simulink model "Two_Zone_MVDC_12pulse_ACDC_degradation"  (R2020b)
settings: Solver=FixedStepAuto  StartTime=0.0  StopTime=40  FixedStep=TsELEC  MaxStep=1  RelTol=1e-3  EnableMultiTasking=on
InitFcn:
  | TsELEC = 1e-4;
  | Ts = 1e-4;
undefined symbols (not defined in the file): DiscIntNeverNeededParam, droop1, droop2, GABDA, GABDB, GBBDA, GBBDB, GPMMA, GPPMB, GPPMC, SADA, SADB, SADC, SADD, SBDA, SBDB, SBDC, SCDA, SCDB, SCDC, SCDD, SDDA, SDDB, SDDC, SDDD, SDDE
libraries: fl_lib x92, nesl_utility x49, ee_lib x36, powerlib x1, simulink x1
(part 3 of 3)

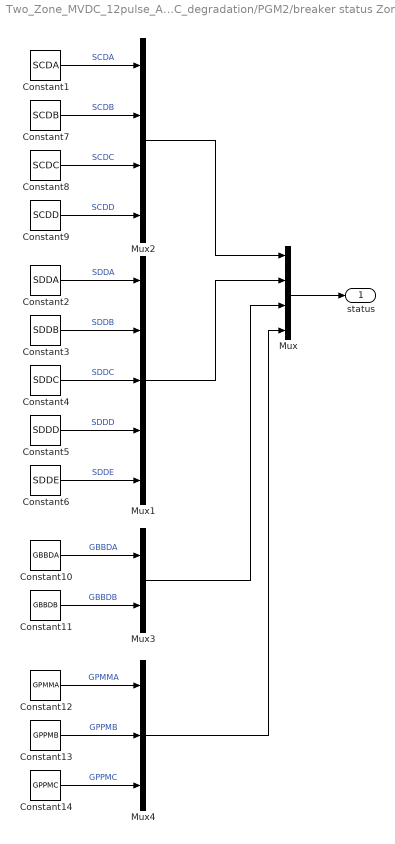
== system Two_Zone_MVDC_12pulse_ACDC_degradation/PGM2/breaker status Zone 2 ==
  Constant1 : Constant  Value=SCDA  SampleTime=Ts
  Constant10 : Constant  Value=GBBDA  SampleTime=Ts
  Constant11 : Constant  Value=GBBDB  SampleTime=Ts
  Constant12 : Constant  Value=GPMMA  SampleTime=Ts
  Constant13 : Constant  Value=GPPMB  SampleTime=Ts
  Constant14 : Constant  Value=GPPMC  SampleTime=Ts
  Constant2 : Constant  Value=SDDA  SampleTime=Ts
  Constant3 : Constant  Value=SDDB  SampleTime=Ts
  Constant4 : Constant  Value=SDDC  VectorParams1D=off  SampleTime=Ts
  Constant5 : Constant  Value=SDDD  SampleTime=Ts
  Constant6 : Constant  Value=SDDE  SampleTime=Ts
  Constant7 : Constant  Value=SCDB  SampleTime=Ts
  Constant8 : Constant  Value=SCDC  SampleTime=Ts
  Constant9 : Constant  Value=SCDD  SampleTime=Ts
  Mux : Mux  Inputs=[4 5 2 3]
  Mux1 : Mux  Inputs=5
  Mux2 : Mux
  Mux3 : Mux  Inputs=2
  Mux4 : Mux  Inputs=3
  status : Outport  VectorParamsAs1DForOutWhenUnconnected=off
  wires:
  Mux/1 -> status/1
  Constant9/1 -> Mux2/4  "SCDD"
  Constant8/1 -> Mux2/3  "SCDC"
  Constant7/1 -> Mux2/2  "SCDB"
  Constant1/1 -> Mux2/1  "SCDA"
  Constant6/1 -> Mux1/5  "SDDE"
  Constant4/1 -> Mux1/3  "SDDC"
  Constant3/1 -> Mux1/2  "SDDB"
  Constant2/1 -> Mux1/1  "SDDA"
  Constant5/1 -> Mux1/4  "SDDD"
  Constant10/1 -> Mux3/1  "GBBDA"
  Constant11/1 -> Mux3/2  "GBBDB"
  Constant12/1 -> Mux4/1  "GPMMA"
  Constant13/1 -> Mux4/2  "GPPMB"
  Constant14/1 -> Mux4/3  "GPPMC"
  Mux2/1 -> Mux/1
  Mux1/1 -> Mux/2
  Mux3/1 -> Mux/3
  Mux4/1 -> Mux/4

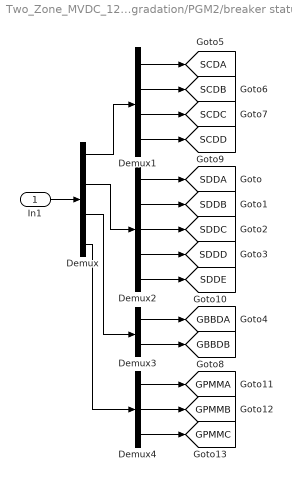
== system Two_Zone_MVDC_12pulse_ACDC_degradation/PGM2/breaker status1 ==
  In1 : Inport
  Demux : Demux  Outputs=[4 5 2 3]
  Demux1 : Demux
  Demux2 : Demux  Outputs=5
  Demux3 : Demux  Outputs=2
  Demux4 : Demux  Outputs=3
  tag scope: GBBDA=global, GBBDB=global, GPMMA=global, GPMMB=global, GPMMC=global, SCDA=global, SCDB=global, SCDC=global, SCDD=global, SDDA=global, SDDB=global, SDDC=global, SDDD=global, SDDE=global
  wires:
  Demux/4 -> Demux4/1
  Demux4/3 -> [GPMMC]
  Demux4/2 -> [GPMMB]
  Demux4/1 -> [GPMMA]
  Demux/3 -> Demux3/1
  Demux3/2 -> [GBBDB]
  Demux3/1 -> [GBBDA]
  Demux/2 -> Demux2/1
  Demux/1 -> Demux1/1
  Demux2/5 -> [SDDE]
  Demux1/4 -> [SCDD]
  Demux1/3 -> [SCDC]
  Demux1/2 -> [SCDB]
  Demux1/1 -> [SCDA]
  In1/1 -> Demux/1
  Demux2/4 -> [SDDD]
  Demux2/3 -> [SDDC]
  Demux2/1 -> [SDDA]
  Demux2/2 -> [SDDB]

== system Two_Zone_MVDC_12pulse_ACDC_degradation/PGM2/voltage droop ==
  droop : Inport
  voltage : Inport  Port=2
  Discrete-Time Integrator : DiscreteIntegrator  gainval=10  InitialCondition=0.9  SampleTime=-1  ICPrevOutput=DiscIntNeverNeededParam  ICPrevScaledInput=DiscIntNeverNeededParam
  Simulink-PS Converter : nesl_utility/Simulink-PS Converter  PhysicalDomain=network_engine_domain  SubClassName=ps_input  LeftPortType=input  RightPortType=output  PseudoPeriodic=off  Frequencies=[]  NoiseDistribution=none  NoiseParameters=[]  Unit=1  AffineConversion=off  FilteringAndDerivatives=provide  SimscapeFilterOrder=1  InputFilterTimeConstant=0.001  UdotUserProvided=0
  Sum : Sum  Inputs=|+-
  Sum1 : Sum  Inputs=|+-
  Vref : Constant
  output : PMIOPort  Side=Right
  wires:
  voltage/1 -> Sum1/2
  Sum1/1 -> Discrete-Time Integrator/1
  Vref/1 -> Sum/1
  droop/1 -> Sum/2
  Sum/1 -> Sum1/1
  Discrete-Time Integrator/1 -> Simulink-PS Converter/1
  connections:
  Simulink-PS Converter/RConn1 -- output/RConn1
